simulink model "model"  (R2021a)
settings: Solver=VariableStepAuto  StartTime=0.0  StopTime=10  RelTol=1e-3
values from neighbouring files (symbols this model uses):
  m = 1    [TP.m]
libraries: roblocks x8, simulink x3
settings Model: Creator=ohvic  LastModifiedBy=ohvic

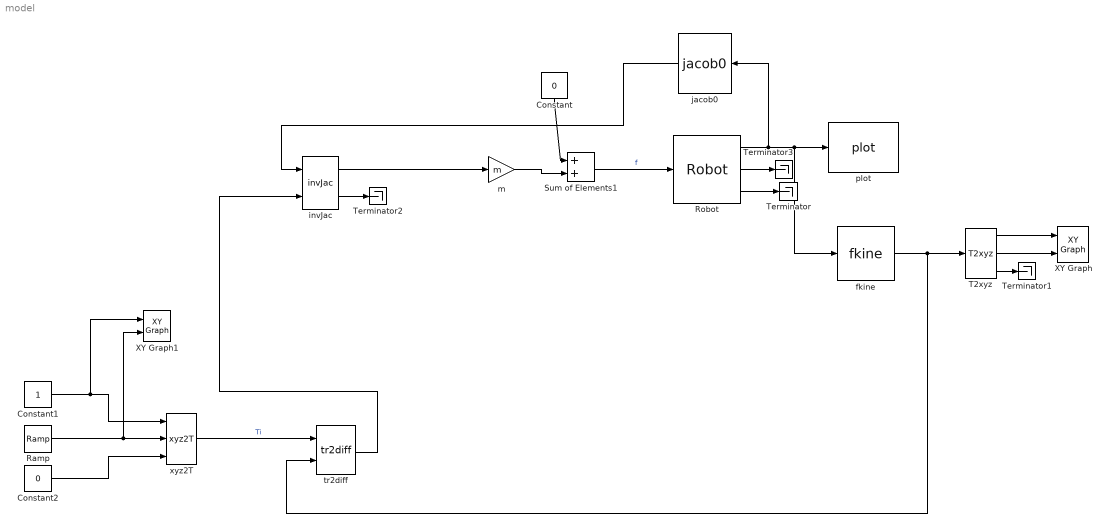
== system model ==
  Constant : Constant  Value=0
  Constant1 : Constant
  Constant2 : Constant  Value=0
  Ramp : simulink/Sources/Ramp  slope=1  start=0  InitialOutput=-1
  Robot : roblocks/Arm/Robot  robot=KR  q0=[0 -pi/2]
  Sum of Elements1 : Sum
  T2xyz : roblocks/Toolbox/T2xyz
  Terminator{,1..3} (4 alike) : Terminator
  XY Graph : simulink/Sinks/XY Graph  xmin=-2  xmax=2  ymin=-2  ymax=2  st=-1
  XY Graph1 : simulink/Sinks/XY Graph  xmin=-1  xmax=1  ymin=-1  ymax=1  st=-1
  fkine : roblocks/Arm/fkine  robot=KR
  invJac : roblocks/Toolbox/invJac
  "jacob0 " : roblocks/Arm/jacob0   robot=KR
  m : Gain  Gain=m
  plot : roblocks/Arm/plot  robot=KR  fps=24  holdplot=on
  tr2diff : roblocks/Toolbox/tr2diff  robot=KR
  xyz2T : roblocks/Toolbox/xyz2T
  wires:
  m/1 -> Sum of Elements1/2
  Sum of Elements1/1 -> Robot/1  "f"
  Robot/1 -> fkine/1, plot/1, "jacob0 "/1
  Constant/1 -> Sum of Elements1/1
  T2xyz/1 -> XY Graph/1
  T2xyz/2 -> XY Graph/2
  fkine/1 -> tr2diff/2, T2xyz/1
  xyz2T/1 -> tr2diff/1  "Ti"
  Constant1/1 -> XY Graph1/1, xyz2T/1
  Constant2/1 -> xyz2T/3
  tr2diff/1 -> invJac/2
  "jacob0 "/1 -> invJac/1
  invJac/1 -> m/1
  Robot/3 -> Terminator/1
  T2xyz/3 -> Terminator1/1
  invJac/2 -> Terminator2/1
  Robot/2 -> Terminator3/1
  Ramp/1 -> XY Graph1/2, xyz2T/2
